simulink model "assignment2"  (R2017b)
settings: Solver=VariableStepAuto  StartTime=0.0  StopTime=10.0  RelTol=1e-3
libraries: hdlsllib x1
settings Model: Creator=Raymond  LastModifiedBy=Raymond

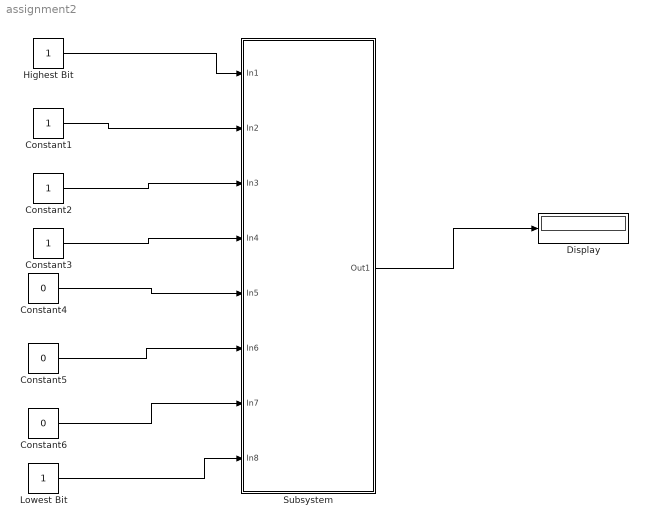
== system assignment2 ==
  Constant1 : Constant  OutDataTypeStr=boolean  SampleTime=-1
  Constant2 : Constant  OutDataTypeStr=boolean  SampleTime=-1
  Constant3 : Constant  OutDataTypeStr=boolean  SampleTime=-1
  Constant4 : Constant  Value=0  OutDataTypeStr=boolean  SampleTime=-1
  Constant5 : Constant  Value=0  OutDataTypeStr=boolean  SampleTime=-1
  Constant6 : Constant  Value=0  OutDataTypeStr=boolean  SampleTime=-1
  Display : Display
  Highest Bit : Constant  OutDataTypeStr=boolean  SampleTime=-1
  Lowest Bit : Constant  OutDataTypeStr=boolean  SampleTime=-1
  Subsystem : Subsystem
  wires:
  Highest Bit/1 -> Subsystem/1(In1)
  Constant1/1 -> Subsystem/2(In2)
  Constant2/1 -> Subsystem/3(In3)
  Constant3/1 -> Subsystem/4(In4)
  Constant4/1 -> Subsystem/5(In5)
  Constant5/1 -> Subsystem/6(In6)
  Constant6/1 -> Subsystem/7(In7)
  Lowest Bit/1 -> Subsystem/8(In8)
  Subsystem/1(Out1) -> Display/1

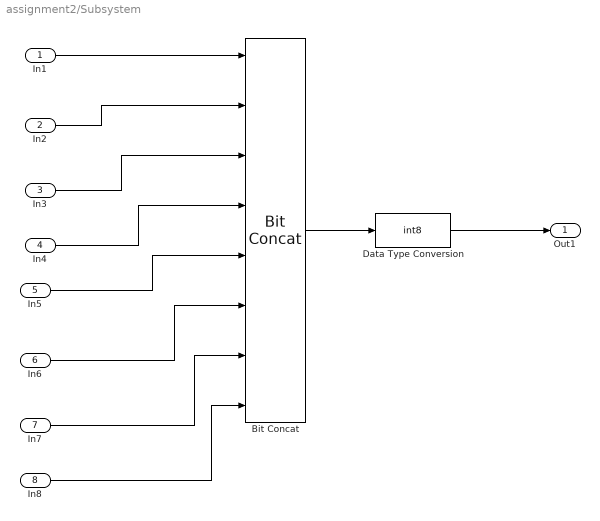
== system assignment2/Subsystem ==
  In1 : Inport
  In2 : Inport  Port=2
  In3 : Inport  Port=3
  In4 : Inport  Port=4
  In5 : Inport  Port=5
  In6 : Inport  Port=6
  In7 : Inport  Port=7
  In8 : Inport  Port=8
  Bit Concat : hdlsllib/Logic and Bit Operations/Bit Concat  numInputs=8
      settings: SourceProductName=HDL Coder  SourceProductBaseCode=HD
  Data Type Conversion : DataTypeConversion  OutDataTypeStr=int8
  Out1 : Outport
  wires:
  Bit Concat/1 -> Data Type Conversion/1
  Data Type Conversion/1 -> Out1/1
  In5/1 -> Bit Concat/5
  In6/1 -> Bit Concat/6
  In1/1 -> Bit Concat/1
  In7/1 -> Bit Concat/7
  In3/1 -> Bit Concat/3
  In4/1 -> Bit Concat/4
  In8/1 -> Bit Concat/8
  In2/1 -> Bit Concat/2
